simulink model "NTCM_G"  (R2021a)
settings: Solver=FixedStepAuto  StartTime=0.0  StopTime=End_Time  FixedStep=Sample_Time  RelTol=1e-3  EnableMultiTasking=on
settings Model: ModifiedByFormat=Francesco Menzione  Creator=Francesco Menzione  LastModifiedBy=Francesco Menzione
settings DataIOCC: ReturnWorkspaceOutputs=off  SignalLoggingName=logsout_new
settings OptimizationCC: UseDivisionForNetSlopeComputation=on  UseFloatMulNetSlope=on  UseSpecifiedMinMax=on  BufferReuse=off  PassReuseOutputArgsAs=Individual arguments  ZeroExternalMemoryAtStartup=off  ZeroInternalMemoryAtStartup=off  EfficientFloat2IntCast=on  LifeSpan=2  EfficientTunableParamExpr=on
settings DebuggingCC: ParameterTunabilityLossMsg=error  AssertControl=DisableAll  SFMachineParentedDataDiag=warning
settings HardwareCC: ProdBitPerPointer=32  ProdBitPerSizeT=32  ProdBitPerPtrDiffT=32  ProdLargestAtomicInteger=LongLong  ProdLargestAtomicFloat=Double  ProdEndianess=BigEndian  ProdWordSize=32  ProdLongLongMode=on  ProdHWDeviceType=Custom Processor->Custom
settings SFSimCC: MATLABDynamicMemAlloc=off
settings RTWCC: SystemTargetFile=ert.tlc  TemplateMakefile=ert_default_tmf  GenerateReport=on  CustomDefine=CheckOn=1  Toolchain=MinGW64 | gmake (64-bit Windows)  BuildConfiguration=Faster Runs  LaunchReport=on  PortableWordSizes=on  CodeExecutionProfiling=on  CodeProfilingInstrumentation=detailed  GenerateTraceReportSl=on  GenerateTraceReportSf=on  GenerateTraceReportEml=on  GenerateWebview=on  GenerateCodeMetricsReport=on  CheckMdlBeforeBuild=Warning
settings CodeAppCC: IgnoreCustomStorageClasses=off  OperatorAnnotations=on  SimulinkDataObjDesc=on  CustomSymbolStrFcn=$M$F  CustomSymbolStrFcnArg=$N$M  CustomSymbolStrBlkIO=lOut_$N$M  InsertBlockDesc=on  SimulinkBlockComments=off
settings ERTTargetCC: TargetLangStandard=C99 (ISO)  UtilityFuncGeneration=Shared location  GenerateSampleERTMain=on  CombineSignalStateStructs=on  SuppressErrorStatus=on  CodeInterfacePackaging=Reusable function  SupportNonFinite=off  SupportComplex=off  RemoveResetFunc=off  ParenthesesLevel=Maximum  CastingMode=Standards  RootIOFormat=Structure reference  ERTSrcFileBannerTemplate=JRCertNTCMG_code_template.cgt  ERTHdrFileBannerTemplate=JRCertNTCMG_code_template.cgt  ERTDataSrcFileTemplate=JRCertNTCMG_code_template.cgt  ERTDataHdrFileTemplate=JRCertNTCMG_code_template.cgt  ERTCustomFileTemplate=example_file_process.tlc  EnableSignedLeftShifts=off  EnableSignedRightShifts=off

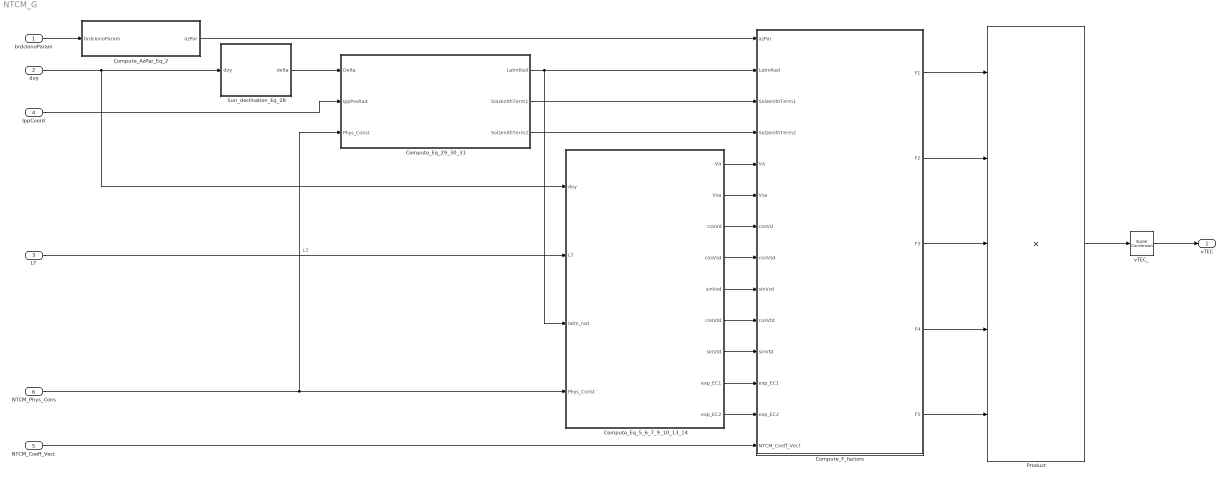
== system NTCM_G ==
  brdcIonoParam : Inport  OutDataTypeStr=double  PortDimensions=[3 1]  SampleTime=[1,0]
  doy : Inport  Port=2  OutDataTypeStr=double  PortDimensions=1  SampleTime=[1,0]
  LT : Inport  Port=3  OutDataTypeStr=double  PortDimensions=1  SampleTime=[1,0]
  IppCoord : Inport  Port=4  OutDataTypeStr=double  PortDimensions=2  SampleTime=[1,0]
  NTCM_Coeff_Vect : Inport  Port=5  OutDataTypeStr=double  PortDimensions=[12 1]
  NTCM_Phys_Cons : Inport  Port=6  OutDataTypeStr=double  PortDimensions=[10 1]
  Compute_AzPar_Eq_2 : Subsystem  Description=|  TreatAsAtomicUnit=on  RTWFcnName=Compute_AzPar_Eq_2
      | <strong> FUNCTION </strong>
      | 
      |    Computation of the proxy measure of the solar activity level (azPar) from the broadcast Ionisation level  parameters ai0,ai1,ai2 (Eq.2)
      | 
      |    @param[in] brdcIonoParam		=> ai0,ai1,ai2 Effective Ionisation Level parameters broadcast in the Galileo Navigation Message
      | 
      |    @param[out] azPar 		=> Proxy measure of the solar activity level
      |    
      | @ingroup NTCM_G
      settings: RTWFcnNameOpts=User specified
  Compute_Eq_29_30_31 : Subsystem  Description=|  TreatAsAtomicUnit=on  RTWFcnName=Compute_Eq_29_30_31
      | <strong> FUNCTION </strong>
      | 
      |    This module computes the dependency of TEC with the solar zenith angle and geomagnetic latitude , see Sec.2.5.6 and 2.5.7 Eq.30,31,32
      | 
      |    @param[in] Delta=> Sun declination Angle [rad]
      |    @param[in] IppCoord =>Pierce Point Coordinates in  Latitude[rad], Longitude[rad]
      |    @param[in] Phys_Const ==> Vector of Pysical Constant see [2]
      | 
      |    @param[out] LatmRad==> geomagnetic latitude
      |    @param[out] SolzenithTerm1==> 1st solar zenith angle 
      |    @param[out] SolzenithTerm2==> 2nd solar zenith angle  
      |    
      |    @ingroup NTCM_G
      settings: RTWFcnNameOpts=User specified
  Compute_Eq_5_6_7_9_10_13_14 : Subsystem  Description=|  TreatAsAtomicUnit=on  RTWFcnName=Compute_Eq_5_6_7_9_10_13_14
      | <strong> FUNCTION </strong>
      | 
      |    This module computes Local time dependency and Seasonal dependency , see Sec.2.4.1 in [1] : Eq.5,6,7,9,10,13,14
      | 
      |    @param[in] Doy => Day of year
      |    @param[in] LT  => Local Time [h]
      |    @param[in] latm_rad => geomagnetic latitude [rad]
      | 
      |    @param[out] Va , Vsa => annual  and semiannual component
      |    @param[out] cosVd, cosVsd, sinVsd, cosVtd, sinVtd, => diurnal, semidiurnal and ter-diurnal  components
      |    @param[out] exp_EC1 => ionisation crests 1st component
      |    @param[out] exp_EC2 => ionisation crests 2nd component
      |    
      | @ingroup NTCM_G
      settings: RTWFcnNameOpts=User specified
  Compute_F_factors : Subsystem  Description=|  TreatAsAtomicUnit=on  RTWFcnName=Compute_F_factors
      | <strong> FUNCTION </strong>
      | 
      |    Compute all dependency contributions ( F factors) and their combination, see Sec.2.4.1
      | 
      |    @param[in] azPar => Proxy measure of the solar activity level
      |    @param[in] LatmRad => Geomagnetic latitude [rad]
      |    @param[in] SolzenithTerm1 => 1st solar zenith angle
      |    @param[in] SolzenithTerm2 => 2nd solar zenith angle
      |    @param[in] Va , Vsa => Annual  and semiannual component
      |    @param[in] cosVd, cosVsd, sinVsd, cosVtd, sinVtd, => diurnal, semidiurnal and ter-diurnal  components
      |    @param[in] exp_EC1 => Ionisation crests 1st component
      |    @param[in] exp_EC2 => Ionisation crests 2nd component
      |    @param[in] NTCM_Coeff_Vect ==> NTCM model coefficients k1,k2,..,k12 (Described in Section 2.4.3)
      | 
      |    @param[out] F1,F2,F3,F4,F5 => Model dependency factors
      | 
      |    @ingroup NTCM_G
      settings: RTWFcnNameOpts=User specified
  Product : Product  Inputs=5
  Sun_declination_Eq_28 : Subsystem  Description=|  TreatAsAtomicUnit=on  RTWFcnName=Sun_declination_Eq_28
      | <strong> FUNCTION </strong>
      | 
      |    This module computes the Sun’s declination for the applicable day (Described in 2.5.5)
      | 
      |    @param[in] doy 		=> Day of the Year
      | 
      |    @param[out] delta_0 		=> Sun's declination [radians]
      |       
      | @ingroup NTCM_G
      settings: RTWFcnNameOpts=User specified
  vTEC_ : SignalConversion  OverrideOpt=off
  vTEC : Outport  OutDataTypeStr=double  PortDimensions=1  SampleTime=[1,0]
  wires:
  NTCM_Phys_Cons/1 -> Compute_Eq_29_30_31/3(Phys_Const), Compute_Eq_5_6_7_9_10_13_14/4(Phys_Const)
  doy/1 -> Sun_declination_Eq_28/1(doy), Compute_Eq_5_6_7_9_10_13_14/1(doy)
  Product/1 -> vTEC_/1
  brdcIonoParam/1 -> Compute_AzPar_Eq_2/1(brdcIonoParam)
  Compute_Eq_29_30_31/1(LatmRad) -> Compute_F_factors/2(LatmRad), Compute_Eq_5_6_7_9_10_13_14/3(latm_rad)
  Sun_declination_Eq_28/1(delta) -> Compute_Eq_29_30_31/1(Delta)
  IppCoord/1 -> Compute_Eq_29_30_31/2(IppPosRad)
  LT/1 -> Compute_Eq_5_6_7_9_10_13_14/2(LT)  "LT"
  Compute_AzPar_Eq_2/1(azPar) -> Compute_F_factors/1(azPar)
  Compute_Eq_29_30_31/2(SolzenithTerm1) -> Compute_F_factors/3(SolzenithTerm1)
  Compute_Eq_29_30_31/3(SolzenithTerm2) -> Compute_F_factors/4(SolzenithTerm2)
  Compute_Eq_5_6_7_9_10_13_14/1(Va) -> Compute_F_factors/5(Va)
  Compute_Eq_5_6_7_9_10_13_14/2(Vsa) -> Compute_F_factors/6(Vsa)
  Compute_Eq_5_6_7_9_10_13_14/3(cosVd) -> Compute_F_factors/7(cosVd)
  Compute_Eq_5_6_7_9_10_13_14/4(cosVsd) -> Compute_F_factors/8(cosVsd)
  Compute_Eq_5_6_7_9_10_13_14/5(sinVsd) -> Compute_F_factors/9(sinVsd)
  Compute_Eq_5_6_7_9_10_13_14/6(cosVtd) -> Compute_F_factors/10(cosVtd)
  Compute_Eq_5_6_7_9_10_13_14/7(sinVtd) -> Compute_F_factors/11(sinVtd)
  Compute_Eq_5_6_7_9_10_13_14/8(exp_EC1) -> Compute_F_factors/12(exp_EC1)
  Compute_Eq_5_6_7_9_10_13_14/9(exp_EC2) -> Compute_F_factors/13(exp_EC2)
  NTCM_Coeff_Vect/1 -> Compute_F_factors/14(NTCM_Coeff_Vect)
  Compute_F_factors/1(F1) -> Product/1
  Compute_F_factors/2(F2) -> Product/2
  Compute_F_factors/3(F3) -> Product/3
  Compute_F_factors/4(F4) -> Product/4
  Compute_F_factors/5(F5) -> Product/5
  vTEC_/1 -> vTEC/1

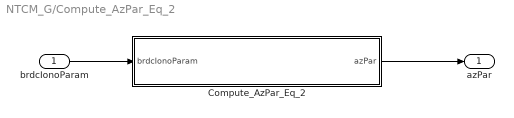
== system NTCM_G/Compute_AzPar_Eq_2 ==
  brdcIonoParam : Inport
  Compute_AzPar_Eq_2 : MATLAB Function  Description=""  RTWFcnName=Compute_F10p7_Eq_2
      settings: FunctionInterfaceSpec=Allow arguments (Optimized)
  azPar : Outport
  wires:
  brdcIonoParam/1 -> Compute_AzPar_Eq_2/1(brdcIonoParam)
  Compute_AzPar_Eq_2/1(azPar) -> azPar/1

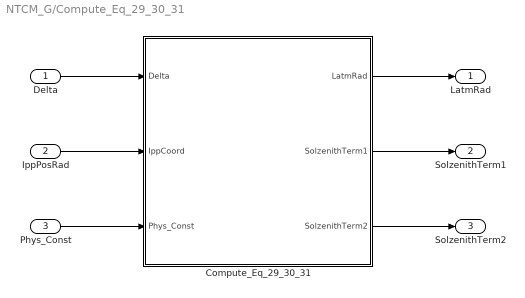
== system NTCM_G/Compute_Eq_29_30_31 ==
  Delta : Inport
  IppPosRad : Inport  Port=2
  Phys_Const : Inport  Port=3
  Compute_Eq_29_30_31 : MATLAB Function  RTWFcnName=Compute_Eq_30_31_32
      settings: FunctionInterfaceSpec=Allow arguments (Optimized)
  LatmRad : Outport
  SolzenithTerm1 : Outport  Port=2
  SolzenithTerm2 : Outport  Port=3
  wires:
  Compute_Eq_29_30_31/2(SolzenithTerm1) -> SolzenithTerm1/1
  Compute_Eq_29_30_31/3(SolzenithTerm2) -> SolzenithTerm2/1
  Phys_Const/1 -> Compute_Eq_29_30_31/3(Phys_Const)
  Delta/1 -> Compute_Eq_29_30_31/1(Delta)
  IppPosRad/1 -> Compute_Eq_29_30_31/2(IppCoord)
  Compute_Eq_29_30_31/1(LatmRad) -> LatmRad/1

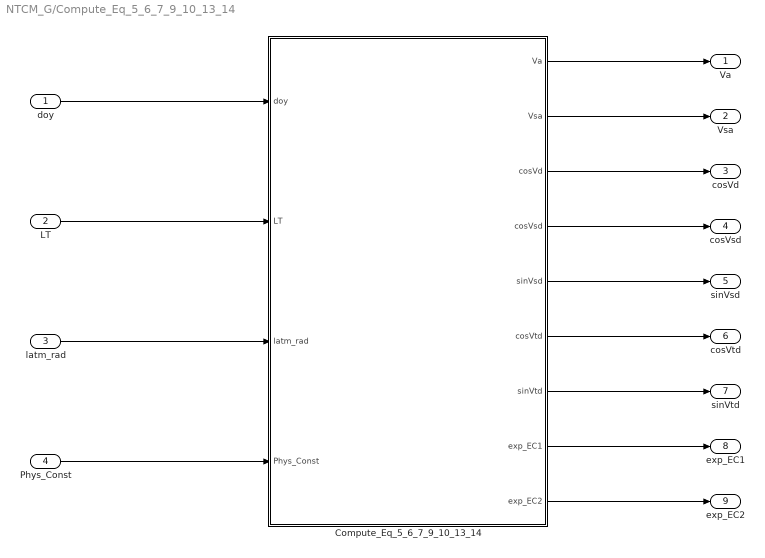
== system NTCM_G/Compute_Eq_5_6_7_9_10_13_14 ==
  doy : Inport
  LT : Inport  Port=2
  latm_rad : Inport  Port=3
  Phys_Const : Inport  Port=4
  Compute_Eq_5_6_7_9_10_13_14 : MATLAB Function  RTWFcnName=Compute_Eq_5_6_7_9_10_13_14
      settings: FunctionInterfaceSpec=Allow arguments (Optimized)
  Va : Outport
  Vsa : Outport  Port=2
  cosVd : Outport  Port=3
  cosVsd : Outport  Port=4
  sinVsd : Outport  Port=5
  cosVtd : Outport  Port=6
  sinVtd : Outport  Port=7
  exp_EC1 : Outport  Port=8
  exp_EC2 : Outport  Port=9
  wires:
  LT/1 -> Compute_Eq_5_6_7_9_10_13_14/2(LT)
  latm_rad/1 -> Compute_Eq_5_6_7_9_10_13_14/3(latm_rad)
  Compute_Eq_5_6_7_9_10_13_14/2(Vsa) -> Vsa/1
  Compute_Eq_5_6_7_9_10_13_14/8(exp_EC1) -> exp_EC1/1
  Compute_Eq_5_6_7_9_10_13_14/5(sinVsd) -> sinVsd/1
  Compute_Eq_5_6_7_9_10_13_14/1(Va) -> Va/1
  Compute_Eq_5_6_7_9_10_13_14/9(exp_EC2) -> exp_EC2/1
  Compute_Eq_5_6_7_9_10_13_14/7(sinVtd) -> sinVtd/1
  Compute_Eq_5_6_7_9_10_13_14/6(cosVtd) -> cosVtd/1
  Phys_Const/1 -> Compute_Eq_5_6_7_9_10_13_14/4(Phys_Const)
  doy/1 -> Compute_Eq_5_6_7_9_10_13_14/1(doy)
  Compute_Eq_5_6_7_9_10_13_14/4(cosVsd) -> cosVsd/1
  Compute_Eq_5_6_7_9_10_13_14/3(cosVd) -> cosVd/1

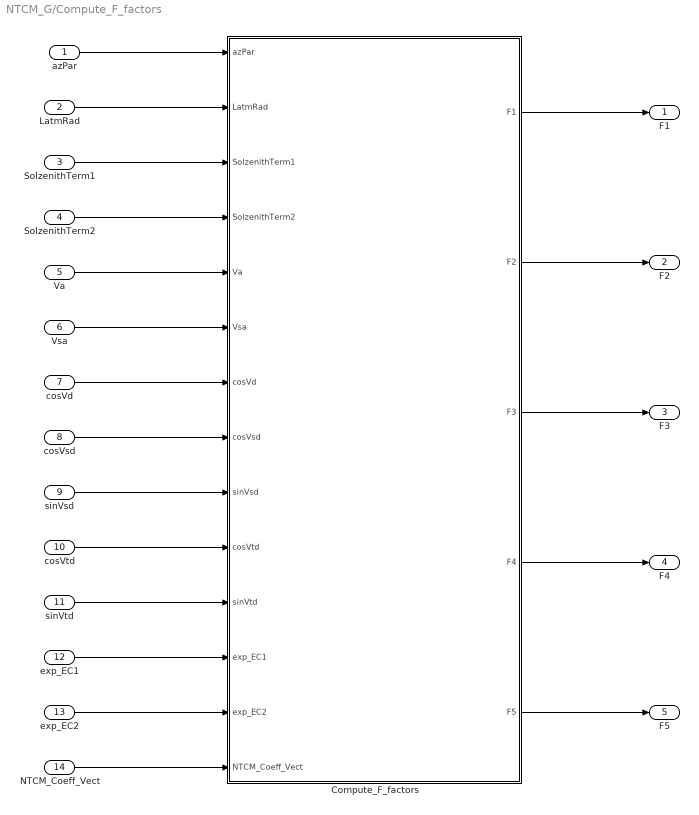
== system NTCM_G/Compute_F_factors ==
  azPar : Inport
  LatmRad : Inport  Port=2
  SolzenithTerm1 : Inport  Port=3
  SolzenithTerm2 : Inport  Port=4
  Va : Inport  Port=5
  Vsa : Inport  Port=6
  cosVd : Inport  Port=7
  cosVsd : Inport  Port=8
  sinVsd : Inport  Port=9
  cosVtd : Inport  Port=10
  sinVtd : Inport  Port=11
  exp_EC1 : Inport  Port=12
  exp_EC2 : Inport  Port=13
  NTCM_Coeff_Vect : Inport  Port=14
  Compute_F_factors : MATLAB Function  RTWFcnName=Compute_F_factors
      settings: FunctionInterfaceSpec=Allow arguments (Optimized)
  F1 : Outport
  F2 : Outport  Port=2
  F3 : Outport  Port=3
  F4 : Outport  Port=4
  F5 : Outport  Port=5
  wires:
  SolzenithTerm1/1 -> Compute_F_factors/3(SolzenithTerm1)
  Va/1 -> Compute_F_factors/5(Va)
  exp_EC1/1 -> Compute_F_factors/12(exp_EC1)
  sinVtd/1 -> Compute_F_factors/11(sinVtd)
  cosVtd/1 -> Compute_F_factors/10(cosVtd)
  cosVsd/1 -> Compute_F_factors/8(cosVsd)
  cosVd/1 -> Compute_F_factors/7(cosVd)
  exp_EC2/1 -> Compute_F_factors/13(exp_EC2)
  Compute_F_factors/3(F3) -> F3/1
  Compute_F_factors/4(F4) -> F4/1
  Vsa/1 -> Compute_F_factors/6(Vsa)
  azPar/1 -> Compute_F_factors/1(azPar)
  Compute_F_factors/5(F5) -> F5/1
  SolzenithTerm2/1 -> Compute_F_factors/4(SolzenithTerm2)
  NTCM_Coeff_Vect/1 -> Compute_F_factors/14(NTCM_Coeff_Vect)
  sinVsd/1 -> Compute_F_factors/9(sinVsd)
  Compute_F_factors/2(F2) -> F2/1
  Compute_F_factors/1(F1) -> F1/1
  LatmRad/1 -> Compute_F_factors/2(LatmRad)

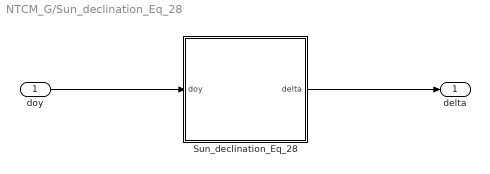
== system NTCM_G/Sun_declination_Eq_28 ==
  doy : Inport
  Sun_declination_Eq_28 : MATLAB Function  Description=""  RTWFcnName=Sun_declination_Eq_29
      settings: FunctionInterfaceSpec=Allow arguments (Optimized)
  delta : Outport
  wires:
  Sun_declination_Eq_28/1(delta) -> delta/1
  doy/1 -> Sun_declination_Eq_28/1(doy)

== matlab function NTCM_G/Compute_AzPar_Eq_2/Compute_AzPar_Eq_2 ==
  data: brdcIonoParam input; azPar output
function azPar = Compute_AzPar_Eq_2(brdcIonoParam)
azPar=0;
azPar         = sqrt(brdcIonoParam(1,1).^2 + ...
                    1633.33*brdcIonoParam(2,1).^2 + ...
                    4802000 * brdcIonoParam(3,1).^2 + ...
                    3266.67 * brdcIonoParam(1,1) .* brdcIonoParam(3,1));

== matlab function NTCM_G/Compute_Eq_29_30_31/Compute_Eq_29_30_31 ==
  data: LatmRad output; SolzenithTerm1 output; SolzenithTerm2 output; Delta input; IppCoord input; Phys_Const input
function [LatmRad,SolzenithTerm1,SolzenithTerm2]= Eq_29_30_31(Delta,IppCoord,Phys_Const)
SolzenithTerm1=0;
SolzenithTerm2=0;
LatmRad=0;

phiIPP = IppCoord(1,1);
lamIPP = IppCoord(2,1);
Pf1=Phys_Const(1,1);

cos_lat_delta    = cos(phiIPP-Delta);

phiGNP_deg=Phys_Const(9,1);
lamGNP_deg=Phys_Const(10,1);
phiGNP     = deg2rad(phiGNP_deg); 
lamGNP     = deg2rad(lamGNP_deg);  

SolzenithTerm1 = cos_lat_delta + Pf1;                                                             % ******  Eq.29                                                                                                                             % ******  Eq.30
SolzenithTerm2    = cos_lat_delta - phiIPP/(pi/2).*sin(Delta);                                    % ******  Eq.30
LatmRad = asin(sin(phiIPP).*sin(phiGNP)+cos(phiIPP).*cos(phiGNP).*cos(lamIPP-lamGNP));            % ******  Eq.31

== matlab function NTCM_G/Compute_F_factors/Compute_F_factors ==
  data: azPar input; LatmRad input; SolzenithTerm1 input; F1 output; SolzenithTerm2 input; Va input; Vsa input; cosVd input; cosVsd input; sinVsd input; cosVtd input; sinVtd input; exp_EC1 input; exp_EC2 input; F2 output; F3 output; NTCM_Coeff_Vect input; F4 output; F5 output
function [F1,F2,F3,F4,F5] = ComputeF_Factors(azPar,LatmRad, SolzenithTerm1,SolzenithTerm2,...
    Va,Vsa,cosVd,cosVsd,sinVsd,cosVtd,sinVtd,exp_EC1,exp_EC2,...
    NTCM_Coeff_Vect)
%#codegen
F1=0;
F2=0;
F3=0;
F4=0;
F5=0;

F1 = SolzenithTerm1 + SolzenithTerm2.*(NTCM_Coeff_Vect(1,1)*cosVd+NTCM_Coeff_Vect(2,1)*cosVsd+NTCM_Coeff_Vect(3,1)*sinVsd+NTCM_Coeff_Vect(4,1)*cosVtd+NTCM_Coeff_Vect(5,1)*sinVtd);       % ******  Eq.4
F2 = 1 + NTCM_Coeff_Vect(6,1).*cos(Va)+NTCM_Coeff_Vect(7,1).*cos(Vsa);                                                               % ******  Eq.8;
F3 = 1 + NTCM_Coeff_Vect(8,1).*cos(LatmRad);                                                                      % ******  Eq.11
F4 = 1 + NTCM_Coeff_Vect(9,1).*exp_EC1+NTCM_Coeff_Vect(10,1).*exp_EC2;                                                               % ******  Eq.12
F5 = NTCM_Coeff_Vect(11,1) + NTCM_Coeff_Vect(12,1).*azPar;                                                                           % ******  Eq.15
  
    
end

== matlab function NTCM_G/Compute_Eq_5_6_7_9_10_13_14/Compute_Eq_5_6_7_9_10_13_14 ==
  data: doy input; LT input; Va output; latm_rad input; Vsa output; cosVd output; Phys_Const input; cosVsd output; sinVsd output; cosVtd output; sinVtd output; exp_EC1 output; exp_EC2 output
function [Va,Vsa,cosVd,cosVsd,sinVsd,cosVtd,sinVtd,exp_EC1,exp_EC2]= ...
    Compute_Eq_5_6_7_9_10_13_14(doy,LT,latm_rad,Phys_Const)

% ****** init
Va=0;
Vsa=0;
cosVd=0;
cosVsd=0;
sinVsd=0;
cosVtd=0;
sinVtd=0;
exp_EC1=0;
exp_EC2=0;

% ****** const
LTd=Phys_Const(2,1);
phi_c1=Phys_Const(5,1);
phi_c2=Phys_Const(6,1);
sigma_c1=Phys_Const(7,1);
sigma_c2=Phys_Const(8,1);
doy_DAV=Phys_Const(3,1);
doy_DSAV=Phys_Const(4,1);

% ******  Eq.5
Vd     = 2*pi*(LT-LTd)/24; 
% ******  Eq.6
Vsd    = 2*pi*LT/12;         
% ******  Eq.7
Vtd    = 2*pi*LT/8;     
% ******  Eq.9
Va     = 2*pi*(doy-doy_DAV)/365.25;
% ******  Eq.10
Vsa    = 4*pi*(doy-doy_DSAV)/365.25;                                                             

cosVd  = cos(Vd);
cosVsd = cos(Vsd);
sinVsd = sin(Vsd);
cosVtd = cos(Vtd);
sinVtd = sin(Vtd);


latm_deg=rad2deg(latm_rad);
EC1 = -(latm_deg-phi_c1)^2/2/sigma_c1^2;                                                         % ******  Eq.13
EC2 = -(latm_deg-phi_c2)^2/2/sigma_c2^2;                                                         % ******  Eq.14
exp_EC1 = exp(EC1);
exp_EC2 = exp(EC2);

== matlab function NTCM_G/Sun_declination_Eq_28/Sun_declination_Eq_28 ==
  data: doy input; delta output
function delta = Sun_declination_Eq_28(doy)
delta=0;
delta = 23.44*sin(0.9856*(doy-80.7)*pi/180)*pi/180;                                            % ******  Eq.28
